simulink model "model"  (R2013a)
settings: Solver=ode45  StartTime=0.0  StopTime=10.0  RelTol=1e-3
values from neighbouring files (symbols this model uses):
  a = 2    [skrypt.m]
  omega = 10    [skrypt.m]
settings Model: Creator=L13-4  LastModifiedBy=Dawid Perdek
settings DataIOCC: SignalLoggingSaveFormat=ModelDataLogs
settings DebuggingCC: UnderspecifiedInitializationDetection=Simplified  MultiTaskDSMMsg=warning  MultiTaskCondExecSysMsg=none  StateNameClashWarn=none  StrictBusMsg=ErrorOnBusTreatedAsVector
settings RTWCC: IncludeERTFirstTime=on
settings GRTTargetCC: CodeReplacementLibrary=None  CPPClassGenCompliant=on

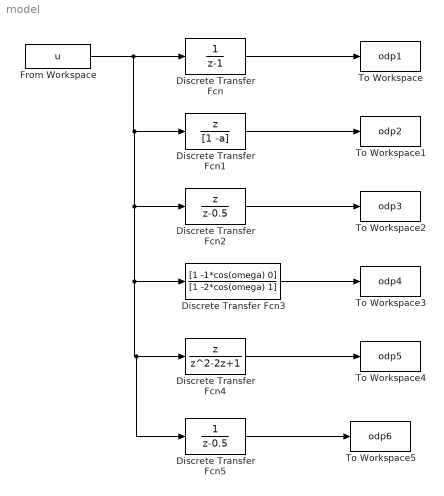
== system model ==
  Discrete Transfer Fcn : DiscreteTransferFcn  Denominator=[1 -1]  SampleTime=0.1
  Discrete Transfer Fcn1 : DiscreteTransferFcn  Numerator=[1 0]  Denominator=[1 -a]  SampleTime=0.1
  Discrete Transfer Fcn2 : DiscreteTransferFcn  Numerator=[1 0]  Denominator=[1 -0.5]  SampleTime=0.1
  Discrete Transfer Fcn3 : DiscreteTransferFcn  Numerator=[1 -1*cos(omega) 0]  Denominator=[1 -2*cos(omega) 1]  SampleTime=0.1
  Discrete Transfer Fcn4 : DiscreteTransferFcn  Numerator=[1 0]  Denominator=[1 -2 1]  SampleTime=0.1
  Discrete Transfer Fcn5 : DiscreteTransferFcn  Denominator=[1 -0.5]  SampleTime=0.1
  From Workspace : FromWorkspace  VariableName=u  SampleTime=0
  To Workspace : ToWorkspace  VariableName=odp1  SampleTime=-1
  To Workspace1 : ToWorkspace  VariableName=odp2  SampleTime=-1
  To Workspace2 : ToWorkspace  VariableName=odp3  SampleTime=-1
  To Workspace3 : ToWorkspace  VariableName=odp4  SampleTime=-1
  To Workspace4 : ToWorkspace  VariableName=odp5  SampleTime=-1
  To Workspace5 : ToWorkspace  VariableName=odp6  SampleTime=-1
  wires:
  From Workspace/1 -> Discrete Transfer Fcn5/1, Discrete Transfer Fcn4/1, Discrete Transfer Fcn3/1, Discrete Transfer Fcn2/1, Discrete Transfer Fcn1/1, Discrete Transfer Fcn/1
  Discrete Transfer Fcn/1 -> To Workspace/1
  Discrete Transfer Fcn1/1 -> To Workspace1/1
  Discrete Transfer Fcn2/1 -> To Workspace2/1
  Discrete Transfer Fcn3/1 -> To Workspace3/1
  Discrete Transfer Fcn4/1 -> To Workspace4/1
  Discrete Transfer Fcn5/1 -> To Workspace5/1
